simulink model "seldom"  (R2024a)
settings: Solver=FixedStepAuto  StartTime=0.0  StopTime=10.0  FixedStep=framePeriod_s  RelTol=1e-3
undefined symbols (not defined in the file): Aircraft, DiscIntNeverNeededParam, framePeriod_s
libraries: simulink x6, sharedtransform x2, slpidlib x2, matrix_library x1
(part 1 of 2)
settings Model: Creator=brian  LastModifiedBy=joshb
settings SolverCC: AlgebraicLoopSolver=TrustRegion
settings OptimizationCC: DefaultParameterBehavior=Inlined  GainParamInheritBuiltInType=on  UseFloatMulNetSlope=on  DefaultUnderspecifiedDataType=single  StrengthReduction=on  ExpressionFolding=off  BitwiseOrLogicalOp=Bitwise operator  PassReuseOutputArgsAs=Individual arguments  ActiveStateOutputEnumStorageType=uint16  ZeroExternalMemoryAtStartup=off  ZeroInternalMemoryAtStartup=off  EfficientFloat2IntCast=on  LifeSpan=inf  OptimizeBlockOrder=speed  DifferentSizesBufferReuse=on  EfficientTunableParamExpr=on
settings DebuggingCC: ReadBeforeWriteMsg=EnableAllAsError  WriteAfterWriteMsg=EnableAllAsError  WriteAfterReadMsg=EnableAllAsError  IntegerOverflowMsg=error  ParameterPrecisionLossMsg=none  ParameterTunabilityLossMsg=error  UnconnectedInputMsg=warning  UnconnectedOutputMsg=warning  UnconnectedLineMsg=warning  UniqueDataStoreMsg=error  BusObjectLabelMismatch=error  RootOutportRequireBusObject=error  NonBusSignalsTreatedAsBus=error  SFInvalidInputDataAccessInChartInitDiag=error  SFTransitionOutsideNaturalParentDiag=error  SFUnreachableExecutionPathDiag=error  SFUndirectedBroadcastEventsDiag=error  IntegerSaturationMsg=error
settings HardwareCC: ProdBitPerPointer=32  ProdBitPerSizeT=32  ProdBitPerPtrDiffT=32  ProdLargestAtomicInteger=Long  ProdLargestAtomicFloat=Double  ProdWordSize=32  ProdHWDeviceType=NXP->Cortex-M4  TargetBitPerLong=64  TargetBitPerPointer=64  TargetBitPerSizeT=64  TargetBitPerPtrDiffT=64  TargetLargestAtomicFloat=Float  TargetIntDivRoundTo=Zero  TargetEndianess=LittleEndian  TargetWordSize=64  TargetHWDeviceType=Intel->x86-64 (Linux 64)  ProdEqTarget=off
settings ModelReferenceCC: EnableRefExpFcnMdlSchedulingChecks=on  ModelReferenceNumInstancesAllowed=Single
settings SFSimCC: SimParseCustomCode=off  SimGenImportedTypeDefs=on  MATLABDynamicMemAlloc=off  SimTargetLang=C++
settings SFSimCC: SimUserIncludeDirs=|
  | ../../flight_code/include
  | ../../../ua_spaaro_extra/imu/include
  | ../../../ua_spaaro_extra/gnss/include
  | ../../../ua_spaaro_extra/pres/include
  | ../../../ua_spaaro_extra/sbus/include
  | ../../../ua_spaaro_extra/global_defs/include
settings SFSimCC: SimUserDefines=|
  | SIL
  | __FMU_R_V2__
settings RTWCC: Description=Embedded Coder  SystemTargetFile=ert.tlc  GenCodeOnly=on  TemplateMakefile=ert_default_tmf  GenerateReport=on  RTWVerbose=off  RTWUseSimCustomCode=on  Toolchain=GNU gcc/g++ | gmake (64-bit Linux)  BuildConfiguration=Specify  IncludeHyperlinkInReport=on  LaunchReport=on  TargetLang=C++  GenerateTraceInfo=on  GenerateTraceReport=on  GenerateTraceReportSl=on  GenerateTraceReportSf=on  GenerateTraceReportEml=on  GenerateCodeReplacementReport=on  GPUComputeCapability=3.5  DLArmComputeVersion=19.05
settings RTWCC: CustomInclude=|
  | ../../flight_code/include
  | ../../../ua_spaaro_extra/imu/include
  | ../../../ua_spaaro_extra/gnss/include
  | ../../../ua_spaaro_extra/pres/include
  | ../../../ua_spaaro_extra/sbus/include
  | ../../../ua_spaaro_extra/global_defs/include
settings RTWCC: CustomDefine=|
  | SIL
  | __FMU_R_V2__
settings CodeAppCC: ForceParamTrailComments=on  IgnoreCustomStorageClasses=off  OperatorAnnotations=on  SimulinkDataObjDesc=on  SFDataObjDesc=on  MATLABFcnDesc=on  CustomSymbolStrGlobalVar=rt$N$M  CustomSymbolStrType=$N$M  CustomSymbolStrFcn=$N$M$F  CustomSymbolStrMacro=$N$M  InsertBlockDesc=on  StateflowObjectComments=on  MATLABSourceComments=on  EnableCustomComments=on  InternalIdentifier=Classic  InlinedPrmAccess=Macros  ReqsInCode=on
settings ERTTargetCC: TargetLangStandard=C++03 (ISO)  GenerateFullHeader=off  IncludeMdlTerminateFcn=off  CombineSignalStateStructs=on  SuppressErrorStatus=on  SupportAbsoluteTime=off  CodeInterfacePackaging=C++ class  SupportComplex=off  ParenthesesLevel=Standards  CastingMode=Standards  GenerateSharedConstants=off  ERTHeaderFileRootName=autocode$E  ERTSourceFileRootName=autocode$E  RootIOFormat=Structure reference  ERTCustomFileTemplate=example_file_process.tlc  ERTFilePackagingFormat=Compact  PreserveExpressionOrder=on  PreserveIfCondition=on  ConvertIfToSwitch=off  EnableSignedLeftShifts=off  EnableSignedRightShifts=off  IndentSize=4

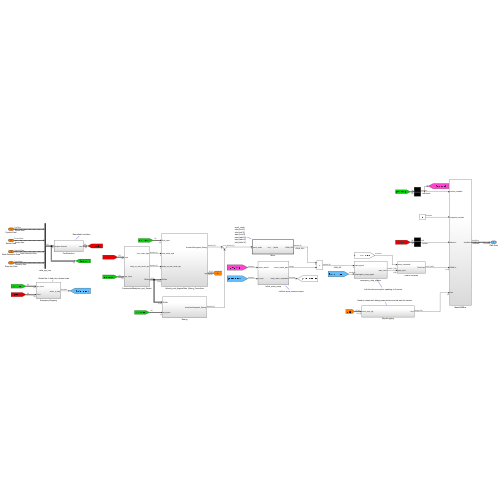
[thumbnail: Simulink's stored preview of the top-level diagram]
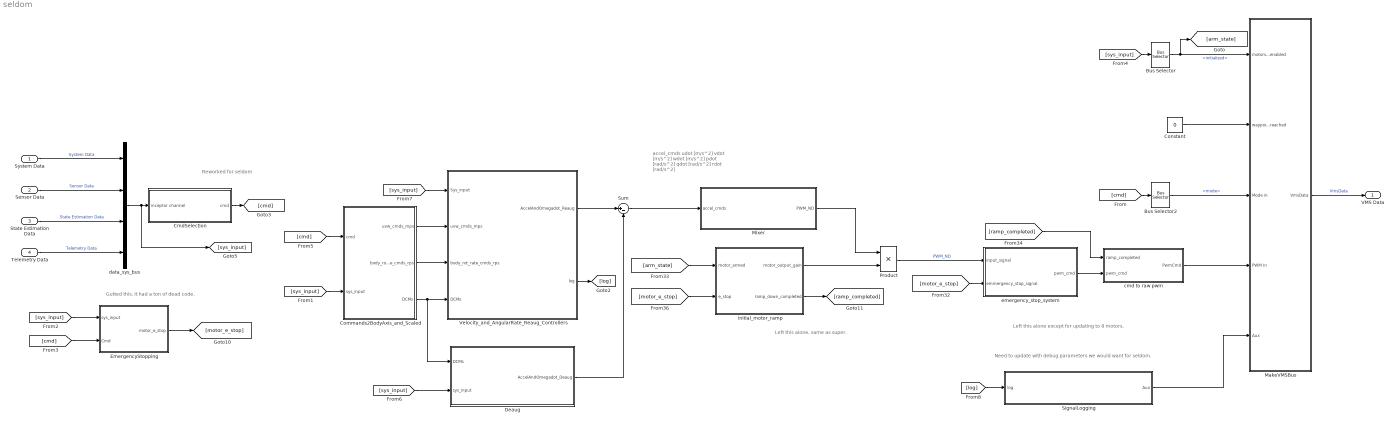
== system seldom ==
  note: accel_cmds
      | udot [m/s^2]
      | vdot [m/s^2]
      | wdot [m/s^2]
      | pdot [rad/s^2]
      | qdot [rad/s^2]
      | rdot [rad/s^2]
  note: Need to update with debug parameters we would want for seldom.
  note: Left this alone, same as super.
  note: Gutted this. It had a ton of dead code.
  note: Reworked for seldom
  note: Left this alone except for updating to 8 motors.
  System Data : Inport  OutDataTypeStr=Bus: SysData  SampleTime=framePeriod_s  BusOutputAsStruct=on
  Sensor Data : Inport  Port=2  OutDataTypeStr=Bus: SensorData  SampleTime=framePeriod_s  BusOutputAsStruct=on
  State Estimation Data : Inport  Port=3  OutDataTypeStr=Bus: StateEstData  SampleTime=framePeriod_s  BusOutputAsStruct=on
  Telemetry Data : Inport  Port=4  OutDataTypeStr=Bus: TelemData  SampleTime=framePeriod_s  BusOutputAsStruct=on
  Bus Selector : BusSelector  OutputSignals=State Estimation Data.bfs_ins.initialized
  Bus Selector2 : BusSelector  OutputSignals=mode
  CmdSelection : Subsystem
  Commands2BodyAxis_and_Scaled : Subsystem
  Constant : Constant  Value=0  OutDataTypeStr=boolean
  Deaug : Subsystem
  EmergencyStopping : Subsystem
  MakeVMSBus : Subsystem
  Mixer : Subsystem
  Product : Product
  SignalLogging : Subsystem
  Sum : Sum  Inputs=|+-
  Velocity_and_AngularRate_Reaug_Controllers : Subsystem
  cmd to raw pwm : Subsystem
  data_sys_bus : BusCreator  Inputs=4
  emergency_stop_system : Subsystem
  initial_motor_ramp : Subsystem
  VMS Data : Outport  OutDataTypeStr=Bus: VmsData  SampleTime=framePeriod_s  BusOutputAsStruct=on
  wires:
  CmdSelection/1(cmd) -> [cmd]
  data_sys_bus/1 -> CmdSelection/1(inceptor channel), [sys_input]
  Velocity_and_AngularRate_Reaug_Controllers/1(AccelAndOmegadot_Reaug) -> Sum/1
  Mixer/1(PWM_ND) -> Product/1
  MakeVMSBus/1(VmsData) -> VMS Data/1  "VmsData"
  cmd to raw pwm/1(PwmCmd) -> MakeVMSBus/4(PWM In)
  [ramp_completed] -> cmd to raw pwm/1(ramp_completed)
  [cmd] -> EmergencyStopping/2(Cmd)
  emergency_stop_system/1(pwm_cmd) -> cmd to raw pwm/2(pwm_cmd)
  [motor_e_stop] -> emergency_stop_system/2(emmergency_stop_signal)
  EmergencyStopping/1(motor_e_stop) -> [motor_e_stop]
  initial_motor_ramp/1(motor_output_gain) -> Product/2
  [motor_e_stop] -> initial_motor_ramp/2(e_stop)
  [arm_state] -> initial_motor_ramp/1(motor_armed)
  Product/1 -> emergency_stop_system/1(input_signal)  "PWM_ND"
  initial_motor_ramp/2(ramp_down_completed) -> [ramp_completed]
  System Data/1 -> data_sys_bus/1  "System Data"
  Sensor Data/1 -> data_sys_bus/2  "Sensor Data"
  Telemetry Data/1 -> data_sys_bus/4  "Telemetry Data"
  [sys_input] -> EmergencyStopping/1(sys_input)
  Bus Selector2/1 -> MakeVMSBus/3(Mode in)  "<mode>"
  Constant/1 -> MakeVMSBus/2(waypoint_reached)
  Bus Selector/1 -> MakeVMSBus/1(motors_enabled), [arm_state]  "<initialized>"
  State Estimation Data/1 -> data_sys_bus/3  "State Estimation Data"
  [sys_input] -> Bus Selector/1
  [cmd] -> Bus Selector2/1
  SignalLogging/1(Aux) -> MakeVMSBus/5(Aux)
  Sum/1 -> Mixer/1(accel_cmds)
  [cmd] -> Commands2BodyAxis_and_Scaled/1(cmd)
  [sys_input] -> Commands2BodyAxis_and_Scaled/2(sys_input)
  Commands2BodyAxis_and_Scaled/3(DCMs) -> Deaug/1(DCMs), Velocity_and_AngularRate_Reaug_Controllers/4(DCMs)
  [sys_input] -> Deaug/2(sys_input)
  Deaug/1(AccelAndOmegadot_Deaug) -> Sum/2
  [sys_input] -> Velocity_and_AngularRate_Reaug_Controllers/1(Sys_input)
  Commands2BodyAxis_and_Scaled/1(uvw_cmds_mps) -> Velocity_and_AngularRate_Reaug_Controllers/2(uvw_cmds_mps)
  Commands2BodyAxis_and_Scaled/2(body_rot_rate_cmds_rps) -> Velocity_and_AngularRate_Reaug_Controllers/3(body_rot_rate_cmds_rps)
  Velocity_and_AngularRate_Reaug_Controllers/2(log) -> [log]
  [log] -> SignalLogging/1(log)

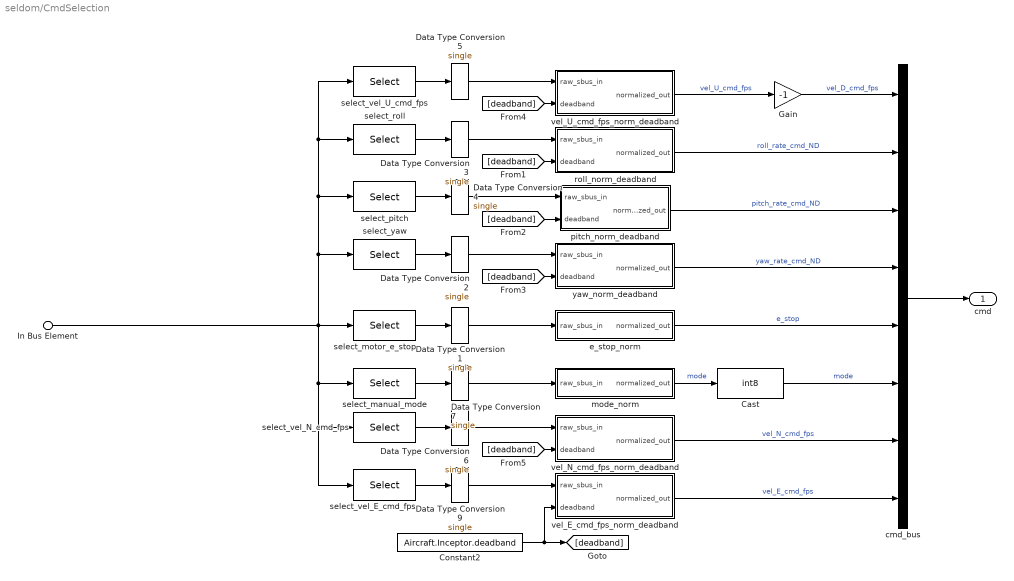
== system seldom/CmdSelection ==
  In Bus Element : Inport  PortName=inceptor channel  Element=Sensor Data.inceptor.ch
  Cast : DataTypeConversion  OutDataTypeStr=int8  SaturateOnIntegerOverflow=off  RndMeth=Floor
  Constant2 : Constant  Value=Aircraft.Inceptor.deadband
  Data Type Conversion{1..7,9} (8 alike) : DataTypeConversion  OutDataTypeStr=single  SaturateOnIntegerOverflow=off  RndMeth=Floor
  Gain : Gain  Gain=-1
  cmd_bus : BusCreator  Inputs=8
  e_stop_norm : Subsystem
  mode_norm : Subsystem
  pitch_norm_deadband : Subsystem
  roll_norm_deadband : Subsystem
  select_manual_mode : Selector  IndexOptions=Index vector (dialog)  Indices=Aircraft.Inceptor.mode  OutputSizes=1
  select_motor_e_stop : Selector  IndexOptions=Index vector (dialog)  Indices=Aircraft.Inceptor.throttle_e_stop  OutputSizes=1
  select_pitch : Selector  IndexOptions=Index vector (dialog)  Indices=Aircraft.Inceptor.pitch_rate  OutputSizes=1
  select_roll : Selector  IndexOptions=Index vector (dialog)  Indices=Aircraft.Inceptor.roll_rate  OutputSizes=1
  select_vel_E_cmd_fps : Selector  IndexOptions=Index vector (dialog)  Indices=Aircraft.Inceptor.vel_E_cmd_fps  OutputSizes=1
  select_vel_N_cmd_fps : Selector  IndexOptions=Index vector (dialog)  Indices=Aircraft.Inceptor.vel_N_cmd_fps  OutputSizes=1
  select_vel_U_cmd_fps : Selector  IndexOptions=Index vector (dialog)  Indices=Aircraft.Inceptor.vel_U_cmd_fps  OutputSizes=1
  select_yaw : Selector  IndexOptions=Index vector (dialog)  Indices=Aircraft.Inceptor.yaw_rate  OutputSizes=1
  vel_E_cmd_fps_norm_deadband : Subsystem
  vel_N_cmd_fps_norm_deadband : Subsystem
  vel_U_cmd_fps_norm_deadband : Subsystem
  yaw_norm_deadband : Subsystem
  cmd : Outport
  wires:
  select_pitch/1 -> Data Type Conversion4/1
  select_yaw/1 -> Data Type Conversion2/1
  Data Type Conversion2/1 -> yaw_norm_deadband/1(raw_sbus_in)
  select_vel_U_cmd_fps/1 -> Data Type Conversion5/1
  Data Type Conversion4/1 -> pitch_norm_deadband/1(raw_sbus_in)
  cmd_bus/1 -> cmd/1
  Data Type Conversion3/1 -> roll_norm_deadband/1(raw_sbus_in)
  Data Type Conversion5/1 -> vel_U_cmd_fps_norm_deadband/1(raw_sbus_in)
  select_roll/1 -> Data Type Conversion3/1
  In Bus Element/1 -> select_vel_E_cmd_fps/1, select_vel_N_cmd_fps/1, select_manual_mode/1, select_vel_U_cmd_fps/1, select_roll/1, select_pitch/1, select_yaw/1, select_motor_e_stop/1
  Data Type Conversion1/1 -> e_stop_norm/1(raw_sbus_in)
  select_motor_e_stop/1 -> Data Type Conversion1/1
  select_vel_N_cmd_fps/1 -> Data Type Conversion6/1
  Data Type Conversion6/1 -> vel_N_cmd_fps_norm_deadband/1(raw_sbus_in)
  Data Type Conversion7/1 -> mode_norm/1(raw_sbus_in)
  select_manual_mode/1 -> Data Type Conversion7/1
  select_vel_E_cmd_fps/1 -> Data Type Conversion9/1
  Data Type Conversion9/1 -> vel_E_cmd_fps_norm_deadband/1(raw_sbus_in)
  Gain/1 -> cmd_bus/1  "vel_D_cmd_fps"
  pitch_norm_deadband/1(normalized_out) -> cmd_bus/3  "pitch_rate_cmd_ND"
  roll_norm_deadband/1(normalized_out) -> cmd_bus/2  "roll_rate_cmd_ND"
  yaw_norm_deadband/1(normalized_out) -> cmd_bus/4  "yaw_rate_cmd_ND"
  e_stop_norm/1(normalized_out) -> cmd_bus/5  "e_stop"
  mode_norm/1(normalized_out) -> Cast/1  "mode"
  vel_N_cmd_fps_norm_deadband/1(normalized_out) -> cmd_bus/7  "vel_N_cmd_fps"
  vel_E_cmd_fps_norm_deadband/1(normalized_out) -> cmd_bus/8  "vel_E_cmd_fps"
  [deadband] -> roll_norm_deadband/2(deadband)
  [deadband] -> vel_U_cmd_fps_norm_deadband/2(deadband)
  [deadband] -> pitch_norm_deadband/2(deadband)
  [deadband] -> yaw_norm_deadband/2(deadband)
  [deadband] -> vel_N_cmd_fps_norm_deadband/2(deadband)
  Constant2/1 -> vel_E_cmd_fps_norm_deadband/2(deadband), [deadband]
  vel_U_cmd_fps_norm_deadband/1(normalized_out) -> Gain/1  "vel_U_cmd_fps"
  Cast/1 -> cmd_bus/6  "mode"

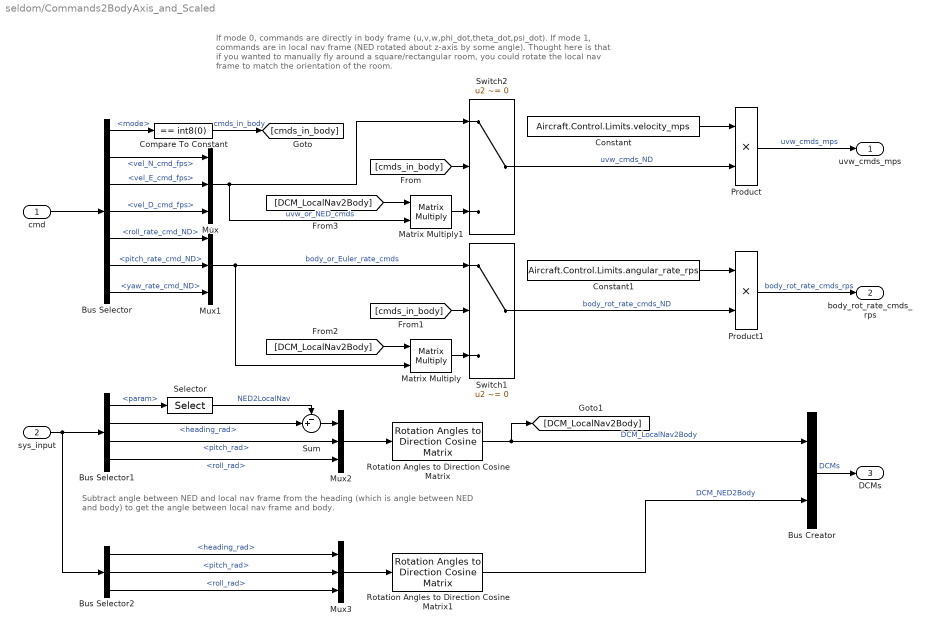
== system seldom/Commands2BodyAxis_and_Scaled ==
  note: Subtract angle between NED and local nav frame from the heading (which is angle between NED and body) to get the angle between local nav frame and body.
  note: If mode 0, commands are directly in body frame (u,v,w,phi_dot,theta_dot,psi_dot).
      | If mode 1, commands are in local nav frame (NED rotated about z-axis by some angle).
      |     Thought here is that if you wanted to manually fly around a square/rectangular room, you could rotate the local nav frame to match the orientation of the room.
  cmd : Inport
  sys_input : Inport  Port=2
  Bus Creator : BusCreator  Inputs=2
  Bus Selector : BusSelector  OutputSignals=mode,vel_N_cmd_fps,vel_E_cmd_fps,vel_D_cmd_fps,roll_rate_cmd_ND,pitch_rate_cmd_ND,yaw_rate_cmd_ND
  Bus Selector1 : BusSelector  OutputSignals=Telemetry Data.param,State Estimation Data.bfs_ins.heading_rad,State Estimation Data.bfs_ins.pitch_rad,State Estimation Data.bfs_ins.roll_rad
  Bus Selector2 : BusSelector  OutputSignals=State Estimation Data.bfs_ins.heading_rad,State Estimation Data.bfs_ins.pitch_rad,State Estimation Data.bfs_ins.roll_rad
  Compare To Constant : simulink/Logic and Bit Operations/Compare To Constant  relop===  const=int8(0)  OutDataTypeStr=boolean
  Constant : Constant  Value=Aircraft.Control.Limits.velocity_mps
  Constant1 : Constant  Value=Aircraft.Control.Limits.angular_rate_rps
  Matrix Multiply : Product  Multiplication=Matrix(*)
  Matrix Multiply1 : Product  Multiplication=Matrix(*)
  Mux{,1..3} (4 alike) : Mux  Inputs=3
  Product : Product
  Product1 : Product
  Rotation Angles to Direction Cosine Matrix : sharedtransform/Rotation Angles to Direction Cosine Matrix  rotationOrder=ZYX  aMode=aMode
  Rotation Angles to Direction Cosine Matrix1 : sharedtransform/Rotation Angles to Direction Cosine Matrix  rotationOrder=ZYX  aMode=aMode
  Selector : Selector  InputPortWidth=24  IndexOptions=Index vector (dialog)  Indices=[1]  OutputSizes=1
  Sum : Sum  Inputs=-+|
  Switch1 : Switch  Criteria=u2 ~= 0  SaturateOnIntegerOverflow=off  InputSameDT=off
  Switch2 : Switch  Criteria=u2 ~= 0  SaturateOnIntegerOverflow=off  InputSameDT=off
  uvw_cmds_mps : Outport
  body_rot_rate_cmds_rps : Outport  Port=2
  DCMs : Outport  Port=3
  wires:
  cmd/1 -> Bus Selector/1
  Bus Selector/1 -> Compare To Constant/1  "<mode>"
  Bus Selector/2 -> Mux/1  "<vel_N_cmd_fps>"
  Bus Selector/3 -> Mux/2  "<vel_E_cmd_fps>"
  Bus Selector/4 -> Mux/3  "<vel_D_cmd_fps>"
  Mux/1 -> Switch2/1, Matrix Multiply1/2  "uvw_or_NED_cmds"
  Bus Selector/5 -> Mux1/1  "<roll_rate_cmd_ND>"
  Bus Selector/6 -> Mux1/2  "<pitch_rate_cmd_ND>"
  Bus Selector/7 -> Mux1/3  "<yaw_rate_cmd_ND>"
  Mux1/1 -> Matrix Multiply/2, Switch1/1  "body_or_Euler_rate_cmds"
  Rotation Angles to Direction Cosine Matrix/1 -> Bus Creator/1, [DCM_LocalNav2Body]  "DCM_LocalNav2Body"
  sys_input/1 -> Bus Selector2/1, Bus Selector1/1
  Bus Selector1/2 -> Sum/2  "<heading_rad>"
  Bus Selector1/3 -> Mux2/2  "<pitch_rad>"
  Bus Selector1/4 -> Mux2/3  "<roll_rad>"
  Mux2/1 -> Rotation Angles to Direction Cosine Matrix/1
  Bus Selector1/1 -> Selector/1  "<param>"
  Selector/1 -> Sum/1  "NED2LocalNav"
  Sum/1 -> Mux2/1
  Compare To Constant/1 -> [cmds_in_body]  "cmds_in_body"
  [cmds_in_body] -> Switch2/2
  [cmds_in_body] -> Switch1/2
  [DCM_LocalNav2Body] -> Matrix Multiply/1
  Matrix Multiply/1 -> Switch1/3
  Matrix Multiply1/1 -> Switch2/3
  [DCM_LocalNav2Body] -> Matrix Multiply1/1
  Switch2/1 -> Product/2  "uvw_cmds_ND"
  Switch1/1 -> Product1/2  "body_rot_rate_cmds_ND"
  Product/1 -> uvw_cmds_mps/1  "uvw_cmds_mps"
  Constant/1 -> Product/1
  Product1/1 -> body_rot_rate_cmds_rps/1  "body_rot_rate_cmds_rps"
  Constant1/1 -> Product1/1
  Mux3/1 -> Rotation Angles to Direction Cosine Matrix1/1
  Bus Selector2/1 -> Mux3/1  "<heading_rad>"
  Bus Selector2/2 -> Mux3/2  "<pitch_rad>"
  Bus Selector2/3 -> Mux3/3  "<roll_rad>"
  Rotation Angles to Direction Cosine Matrix1/1 -> Bus Creator/2  "DCM_NED2Body"
  Bus Creator/1 -> DCMs/1  "DCMs"

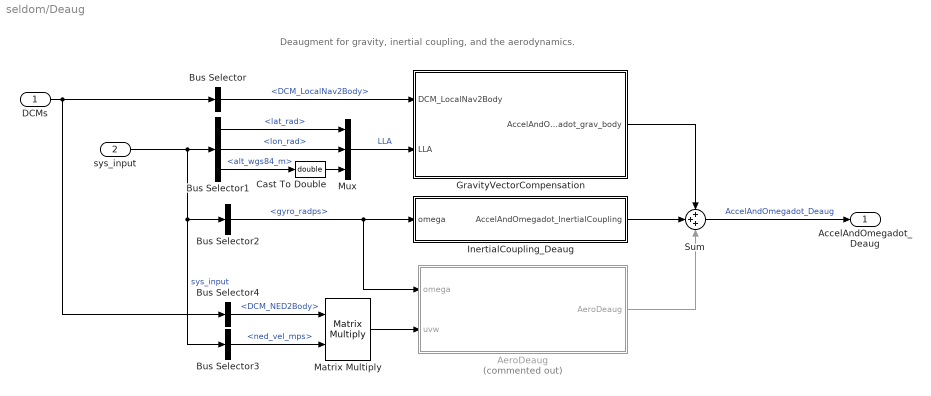
== system seldom/Deaug ==
  note: Deaugment for gravity, inertial coupling, and the aerodynamics.
  DCMs : Inport
  sys_input : Inport  Port=2
  AeroDeaug : Subsystem  Commented=on
  Bus Selector : BusSelector  OutputSignals=DCM_LocalNav2Body
  Bus Selector1 : BusSelector  OutputSignals=Sensor Data.ext_gnss1.lat_rad,Sensor Data.ext_gnss1.lon_rad,Sensor Data.ext_gnss1.alt_wgs84_m
  Bus Selector2 : BusSelector  OutputSignals=Sensor Data.fmu_imu.gyro_radps
  Bus Selector3 : BusSelector  OutputSignals=State Estimation Data.bfs_ins.ned_vel_mps
  Bus Selector4 : BusSelector  OutputSignals=DCM_NED2Body
  Cast To Double : DataTypeConversion  OutDataTypeStr=double  SaturateOnIntegerOverflow=off  RndMeth=Floor
  GravityVectorCompensation : Subsystem
  InertialCoupling_Deaug : Subsystem
  Matrix Multiply : Product  Multiplication=Matrix(*)
  Mux : Mux  Inputs=3
  Sum : Sum  Inputs=+++
  AccelAndOmegadot_Deaug : Outport
  wires:
  Bus Selector1/2 -> Mux/2  "<lon_rad>"
  Bus Selector/1 -> GravityVectorCompensation/1(DCM_LocalNav2Body)  "<DCM_LocalNav2Body>"
  sys_input/1 -> Bus Selector1/1, Bus Selector2/1, Bus Selector3/1  "sys_input"
  Bus Selector1/3 -> Cast To Double/1  "<alt_wgs84_m>"
  GravityVectorCompensation/1(AccelAndOmegadot_grav_body) -> Sum/1
  Mux/1 -> GravityVectorCompensation/2(LLA)  "LLA"
  InertialCoupling_Deaug/1(AccelAndOmegadot_InertialCoupling) -> Sum/2
  Bus Selector1/1 -> Mux/1  "<lat_rad>"
  Bus Selector2/1 -> AeroDeaug/1(omega), InertialCoupling_Deaug/1(omega)  "<gyro_radps>"
  Bus Selector3/1 -> Matrix Multiply/2  "<ned_vel_mps>"
  Bus Selector4/1 -> Matrix Multiply/1  "<DCM_NED2Body>"
  Matrix Multiply/1 -> AeroDeaug/2(uvw)
  AeroDeaug/1(AeroDeaug) -> Sum/3
  Sum/1 -> AccelAndOmegadot_Deaug/1  "AccelAndOmegadot_Deaug"
  Cast To Double/1 -> Mux/3
  DCMs/1 -> Bus Selector4/1, Bus Selector/1

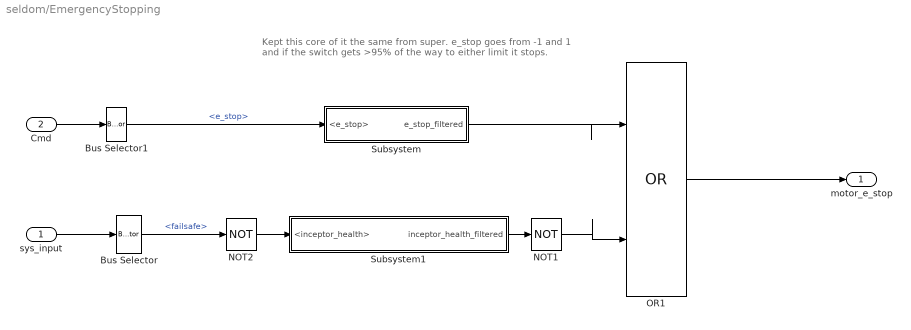
== system seldom/EmergencyStopping ==
  note: Kept this core of it the same from super. e_stop goes from -1 and 1 and if the switch gets >95% of the way to either limit it stops.
  sys_input : Inport
  Cmd : Inport  Port=2
  Bus Selector : BusSelector  OutputSignals=Sensor Data.inceptor.failsafe
  Bus Selector1 : BusSelector  OutputSignals=e_stop
  NOT1 : Logic  Operator=NOT  IconShape=distinctive  AllPortsSameDT=off  OutDataTypeStr=boolean
  NOT2 : Logic  Operator=NOT  IconShape=distinctive  AllPortsSameDT=off  OutDataTypeStr=boolean
  OR1 : Logic  Operator=OR  IconShape=distinctive  AllPortsSameDT=off  OutDataTypeStr=boolean
  Subsystem : Subsystem
  Subsystem1 : Subsystem
  motor_e_stop : Outport
  wires:
  Bus Selector/1 -> NOT2/1  "<failsafe>"
  sys_input/1 -> Bus Selector/1
  Bus Selector1/1 -> Subsystem/1(<e_stop>)  "<e_stop>"
  Cmd/1 -> Bus Selector1/1
  OR1/1 -> motor_e_stop/1
  NOT1/1 -> OR1/2
  Subsystem/1(e_stop_filtered) -> OR1/1
  NOT2/1 -> Subsystem1/1(<inceptor_health>)
  Subsystem1/1(inceptor_health_filtered) -> NOT1/1

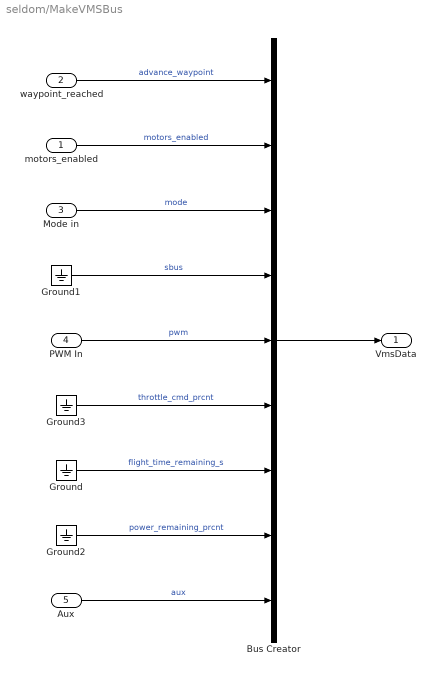
== system seldom/MakeVMSBus ==
  motors_enabled : Inport
  waypoint_reached : Inport  Port=2
  Mode in : Inport  Port=3
  PWM In : Inport  Port=4
  Aux : Inport  Port=5
  Bus Creator : BusCreator  Inputs=9  OutDataTypeStr=Bus: VmsData  NonVirtualBus=on
      settings: InheritFromInputs=off
  Ground{,1..3} (4 alike) : Ground
  VmsData : Outport
  wires:
  Bus Creator/1 -> VmsData/1
  waypoint_reached/1 -> Bus Creator/1  "advance_waypoint"
  motors_enabled/1 -> Bus Creator/2  "motors_enabled"
  Mode in/1 -> Bus Creator/3  "mode"
  Ground1/1 -> Bus Creator/4  "sbus"
  PWM In/1 -> Bus Creator/5  "pwm"
  Ground3/1 -> Bus Creator/6  "throttle_cmd_prcnt"
  Aux/1 -> Bus Creator/9  "aux"
  Ground/1 -> Bus Creator/7  "flight_time_remaining_s"
  Ground2/1 -> Bus Creator/8  "power_remaining_prcnt"

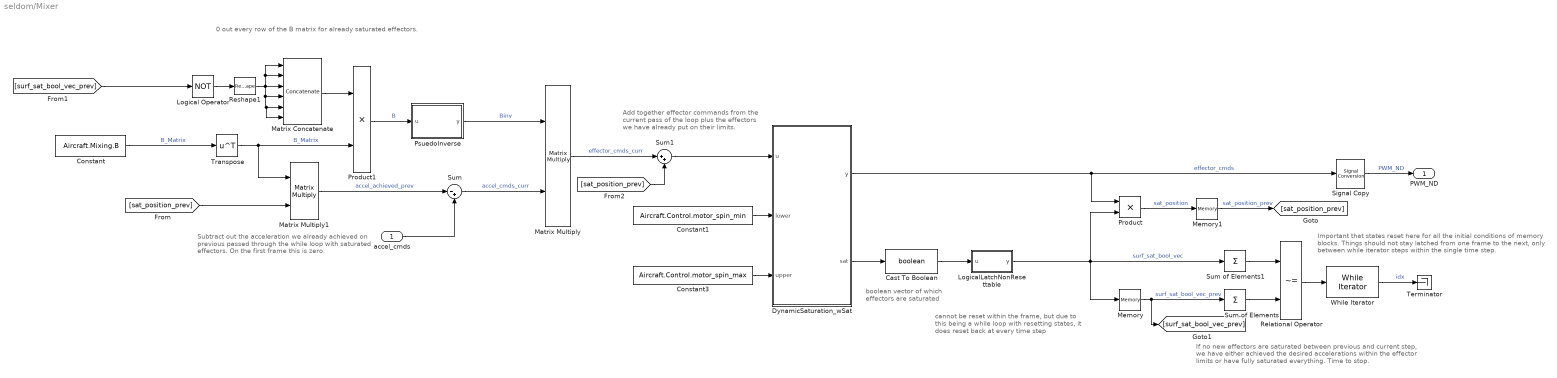
== system seldom/Mixer ==
  note: Add together effector commands from the current pass of the loop plus the effectors we have already put on their limits.
  note: Subtract out the acceleration we already achieved on previous passed through the while loop with saturated effectors. On the first frame this is zero.
  note: 0 out every row of the B matrix for already saturated effectors.
  note: Important that states reset here for all the initial conditions of memory blocks. Things should not stay latched from one frame to the next, only between while iterator steps within the single time step.
  note: If no new effectors are saturated between previous and current step, we have either achieved the desired accelerations within the effector limits or have fully saturated everything. Time to stop.
  note: cannot be reset within the frame, but due to this being a while loop with resetting states, it does reset back at every time step
  note: boolean vector of which effectors are saturated
  accel_cmds : Inport
  Cast To Boolean : DataTypeConversion  OutDataTypeStr=boolean  SaturateOnIntegerOverflow=off  RndMeth=Floor
  Constant : Constant  Value=Aircraft.Mixing.B
  Constant1 : Constant  Value=Aircraft.Control.motor_spin_min  OutDataTypeStr=single
  Constant3 : Constant  Value=Aircraft.Control.motor_spin_max  OutDataTypeStr=single
  DynamicSaturation_wSat : Subsystem
  Logical Operator : Logic  Operator=NOT  AllPortsSameDT=off  OutDataTypeStr=boolean
  LogicalLatchNonResettable : Subsystem
  Matrix Concatenate : Concatenate  NumInputs=6  Mode=Multidimensional array
  Matrix Multiply : Product  Multiplication=Matrix(*)
  Matrix Multiply1 : Product  Multiplication=Matrix(*)
  Memory : Memory  InitialCondition=zeros(1,Aircraft.Motor.nMotor)  InheritSampleTime=on
  Memory1 : Memory  InitialCondition=zeros(1,Aircraft.Motor.nMotor)  InheritSampleTime=on
  Product : Product
  Product1 : Product
  PsuedoInverse : MATLAB Function  TreatAsAtomicUnit=on
  Relational Operator : RelationalOperator  Operator=~=  OutDataTypeStr=boolean  RndMeth=Simplest  InputSameDT=off
  Reshape1 : Reshape  OutputDimensionality=Row vector (2-D)
  Signal Copy : SignalConversion  OverrideOpt=off
  Sum : Sum  Inputs=|-+
  Sum of Elements : Sum  Inputs=+
  Sum of Elements1 : Sum  Inputs=+
  Sum1 : Sum  Inputs=|++
  Terminator : Terminator
  Transpose : Math  Operator=transpose
  While Iterator : WhileIterator  WhileBlockType=do-while  ResetStates=reset  ShowIterationPort=on
  PWM_ND : Outport
  wires:
  Constant/1 -> Transpose/1  "B_Matrix"
  accel_cmds/1 -> Sum/2
  DynamicSaturation_wSat/1(y) -> Product/1, Signal Copy/1  "effector_cmds"
  Constant3/1 -> DynamicSaturation_wSat/3(upper)
  Constant1/1 -> DynamicSaturation_wSat/2(lower)
  Sum1/1 -> DynamicSaturation_wSat/1(u)
  DynamicSaturation_wSat/2(sat) -> Cast To Boolean/1
  Cast To Boolean/1 -> LogicalLatchNonResettable/1(u)
  LogicalLatchNonResettable/1(y) -> Product/2, Sum of Elements1/1, Memory/1  "surf_sat_bool_vec"
  Memory/1 -> Sum of Elements/1, [surf_sat_bool_vec_prev]  "surf_sat_bool_vec_prev"
  Sum of Elements/1 -> Relational Operator/2
  Sum of Elements1/1 -> Relational Operator/1
  Relational Operator/1 -> While Iterator/1
  While Iterator/1 -> Terminator/1  "idx"
  Product/1 -> Memory1/1  "sat_position"
  Memory1/1 -> [sat_position_prev]  "sat_position_prev"
  [sat_position_prev] -> Matrix Multiply1/2
  [surf_sat_bool_vec_prev] -> Logical Operator/1
  Logical Operator/1 -> Reshape1/1
  Reshape1/1 -> Matrix Concatenate/6, Matrix Concatenate/5, Matrix Concatenate/4, Matrix Concatenate/1, Matrix Concatenate/2, Matrix Concatenate/3
  Matrix Concatenate/1 -> Product1/1
  Transpose/1 -> Product1/2, Matrix Multiply1/1  "B_Matrix"
  Product1/1 -> PsuedoInverse/1(u)  "B"
  PsuedoInverse/1(y) -> Matrix Multiply/1  "Binv"
  Matrix Multiply1/1 -> Sum/1  "accel_achieved_prev"
  Sum/1 -> Matrix Multiply/2  "accel_cmds_curr"
  Matrix Multiply/1 -> Sum1/1  "effector_cmds_curr"
  [sat_position_prev] -> Sum1/2
  Signal Copy/1 -> PWM_ND/1  "PWM_ND"

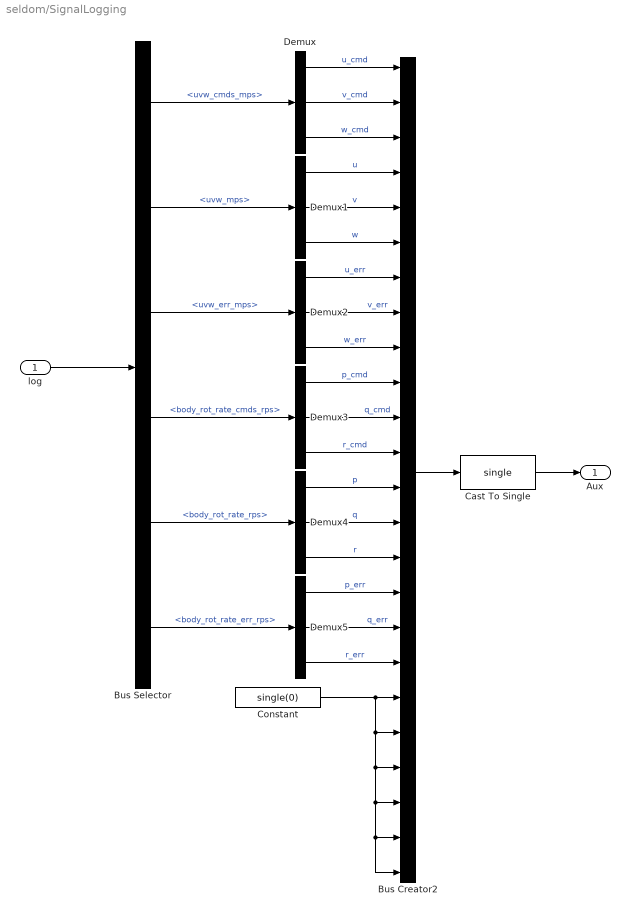
== system seldom/SignalLogging ==
  log : Inport
  Bus Creator2 : BusCreator  Inputs=24
  Bus Selector : BusSelector  OutputSignals=uvw_cmds_mps,uvw_mps,uvw_err_mps,body_rot_rate_cmds_rps,body_rot_rate_rps,body_rot_rate_err_rps
  Cast To Single : DataTypeConversion  OutDataTypeStr=single  SaturateOnIntegerOverflow=off  RndMeth=Floor
  Constant : Constant  Value=single(0)
  Demux{,1..5} (6 alike) : Demux  Outputs=3
  Aux : Outport
  wires:
  Cast To Single/1 -> Aux/1
  Bus Creator2/1 -> Cast To Single/1
  log/1 -> Bus Selector/1
  Bus Selector/6 -> Demux5/1  "<body_rot_rate_err_rps>"
  Demux/1 -> Bus Creator2/1  "u_cmd"
  Demux/2 -> Bus Creator2/2  "v_cmd"
  Demux/3 -> Bus Creator2/3  "w_cmd"
  Demux1/1 -> Bus Creator2/4  "u"
  Demux1/2 -> Bus Creator2/5  "v"
  Demux1/3 -> Bus Creator2/6  "w"
  Demux2/1 -> Bus Creator2/7  "u_err"
  Demux2/2 -> Bus Creator2/8  "v_err"
  Demux2/3 -> Bus Creator2/9  "w_err"
  Demux5/3 -> Bus Creator2/18  "r_err"
  Demux5/2 -> Bus Creator2/17  "q_err"
  Demux5/1 -> Bus Creator2/16  "p_err"
  Demux4/3 -> Bus Creator2/15  "r"
  Demux4/2 -> Bus Creator2/14  "q"
  Demux4/1 -> Bus Creator2/13  "p"
  Demux3/3 -> Bus Creator2/12  "r_cmd"
  Demux3/2 -> Bus Creator2/11  "q_cmd"
  Demux3/1 -> Bus Creator2/10  "p_cmd"
  Bus Selector/2 -> Demux1/1  "<uvw_mps>"
  Bus Selector/1 -> Demux/1  "<uvw_cmds_mps>"
  Bus Selector/3 -> Demux2/1  "<uvw_err_mps>"
  Bus Selector/4 -> Demux3/1  "<body_rot_rate_cmds_rps>"
  Bus Selector/5 -> Demux4/1  "<body_rot_rate_rps>"
  Constant/1 -> Bus Creator2/20, Bus Creator2/21, Bus Creator2/23, Bus Creator2/24, Bus Creator2/22, Bus Creator2/19

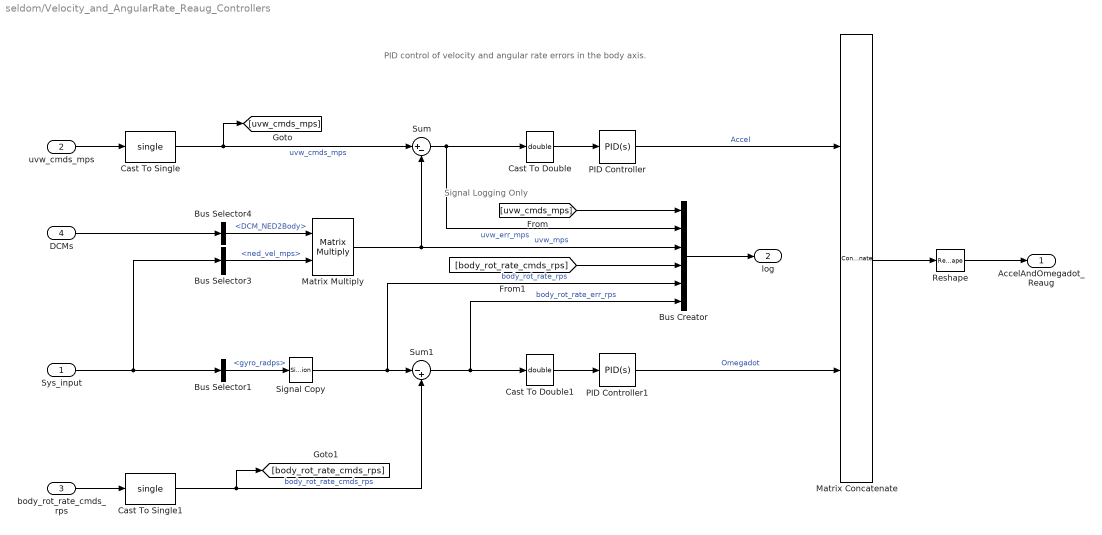
== system seldom/Velocity_and_AngularRate_Reaug_Controllers ==
  note: PID control of velocity and angular rate errors in the body axis.
  note: Signal Logging Only
  Sys_input : Inport
  uvw_cmds_mps : Inport  Port=2
  body_rot_rate_cmds_rps : Inport  Port=3
  DCMs : Inport  Port=4
  Bus Creator : BusCreator  Inputs=6
  Bus Selector1 : BusSelector  OutputSignals=Sensor Data.fmu_imu.gyro_radps
  Bus Selector3 : BusSelector  OutputSignals=State Estimation Data.bfs_ins.ned_vel_mps
  Bus Selector4 : BusSelector  OutputSignals=DCM_NED2Body
  Cast To Double : DataTypeConversion  OutDataTypeStr=double  SaturateOnIntegerOverflow=off  RndMeth=Floor
  Cast To Double1 : DataTypeConversion  OutDataTypeStr=double  SaturateOnIntegerOverflow=off  RndMeth=Floor
  Cast To Single : DataTypeConversion  OutDataTypeStr=single  SaturateOnIntegerOverflow=off  RndMeth=Floor
  Cast To Single1 : DataTypeConversion  OutDataTypeStr=single  SaturateOnIntegerOverflow=off  RndMeth=Floor
  Matrix Concatenate : Concatenate  Mode=Multidimensional array
  Matrix Multiply : Product  Multiplication=Matrix(*)
  PID Controller : slpidlib/PID Controller  Controller=PID  Form=Parallel  TimeDomain=Continuous-time  UseExternalTs=off  SampleTime=-1  IntegratorMethod=Forward Euler  FilterMethod=Forward Euler  ControllerParametersSource=internal  P=1  I=.1  UseKiTs=off  D=.3  UseExternalDerivativeSource=off  N=100  UseFilter=on  TunerSelectOption=Transfer Function Based (PID Tuner App)  InitialConditionSource=internal  InitialConditionForIntegrator=0  InitialConditionForFilter=0  DifferentiatorICPrevScaledInput=0  ExternalReset=none  TrackingMode=off  Kt=1  LimitOutput=off  SatLimitsSource=internal  UpperSaturationLimit=inf  LowerSaturationLimit=-inf  LinearizeAsGain=on  AntiWindupMode=none  Kb=1  LimitIntegrator=off  UpperIntegratorSaturationLimit=inf  LowerIntegratorSaturationLimit=-inf  POutMin=[]  POutMax=[]  IOutMin=[]  IOutMax=[]  DOutMin=[]  DOutMax=[]  NOutMin=[]  NOutMax=[]  SumOutMin=[]  SumOutMax=[]  SaturationOutMin=[]  SaturationOutMax=[]  PParamMin=[]  PParamMax=[]  IParamMin=[]  IParamMax=[]  DParamMin=[]  DParamMax=[]  NParamMin=[]  NParamMax=[]  KbParamMin=[]  KbParamMax=[]  KtParamMin=[]  KtParamMax=[]  KbOutMin=[]  KbOutMax=[]  KtOutMin=[]  KtOutMax=[]  IntegratorOutMin=[]  IntegratorOutMax=[]  FilterOutMin=[]  FilterOutMax=[]  SumI1OutMin=[]  SumI1OutMax=[]  SumI2OutMin=[]  SumI2OutMax=[]  SumI3OutMin=[]  SumI3OutMax=[]  SumI4OutMin=[]  SumI4OutMax=[]  SumDOutMin=[]  SumDOutMax=[]  DifferentiatorOutMin=[]  DifferentiatorOutMax=[]  FilterDiffOutCoefMin=[]  FilterDiffOutCoefMax=[]  ReciprocalOutMin=[]  ReciprocalOutMax=[]  SumDenOutMin=[]  SumDenOutMax=[]  SumNumOutMin=[]  SumNumOutMax=[]  DivideOutMin=[]  DivideOutMax=[]  UdiffTsProdOutMin=[]  UdiffTsProdOutMax=[]  NTsProdOutMin=[]  NTsProdOutMax=[]  UintegralTsProdOutMin=[]  UintegralTsProdOutMax=[]  UngainTsProdOutMin=[]  UngainTsProdOutMax=[]  ClampingZeroOutDataTypeStr=Inherit: Inherit via back propagation  ClampingZeroOutMin=[]  ClampingZeroOutMax=[]  FilterDenConstantOutDataTypeStr=Inherit: Inherit via back propagation  FilterDenConstantOutMin=[]  FilterDenConstantOutMax=[]  PCopyOutDataTypeStr=Inherit: Inherit via back propagation  PCopyOutMin=[]  PCopyOutMax=[]  NCopyOutDataTypeStr=Inherit: Inherit via back propagation  NCopyOutMin=[]  NCopyOutMax=[]  IntegratorContinuousStateAttributes=''  IntegratorStateMustResolveToSignalObject=off  IntegratorRTWStateStorageClass=Auto  FilterContinuousStateAttributes=''  FilterStateMustResolveToSignalObject=off  FilterRTWStateStorageClass=Auto  ParallelPVariant=InternalParameters  IdealPVariant=Disabled  IVariant=InternalParameters  DVariant=InternalParameters  IntegratorVariant=Continuous  SatVariant=Disabled  AWVariant=Passthrough  PCopyVariant=Disabled  TRVariant=Disabled  FdbkBlocksVariant=Forward  IdealPFdbkVariant=Disabled  SatFdbkVariant=Disabled  DerivativeFilterVariant=ContFilter  NVariant=InternalParameters  NCopyVariant=Disabled  FilterICVariant=InternalICsFilter  IntegratorICVariant=InternalICs  ExternalResetVariant=Disabled  TRSumVariant=Passthrough  SumFdbkVariant=Disabled  SumVariant=Sum_PID  TsampFilterVariant=InternalTs  TsampNgainVariant=Passthrough  TsampIntegralVariant=Disabled_SignalSpec  ExternalSaturationOutDataTypeStr=Inherit: Same as second input  DerivativeSourceVariant=ErrorSignal
  PID Controller1 : slpidlib/PID Controller  Controller=PID  Form=Parallel  TimeDomain=Continuous-time  UseExternalTs=off  SampleTime=-1  IntegratorMethod=Forward Euler  FilterMethod=Forward Euler  ControllerParametersSource=internal  P=.5  I=.05  UseKiTs=off  D=.15  UseExternalDerivativeSource=off  N=100  UseFilter=on  TunerSelectOption=Transfer Function Based (PID Tuner App)  InitialConditionSource=internal  InitialConditionForIntegrator=0  InitialConditionForFilter=0  DifferentiatorICPrevScaledInput=0  ExternalReset=none  TrackingMode=off  Kt=1  LimitOutput=off  SatLimitsSource=internal  UpperSaturationLimit=inf  LowerSaturationLimit=-inf  LinearizeAsGain=on  AntiWindupMode=none  Kb=1  LimitIntegrator=off  UpperIntegratorSaturationLimit=inf  LowerIntegratorSaturationLimit=-inf  POutMin=[]  POutMax=[]  IOutMin=[]  IOutMax=[]  DOutMin=[]  DOutMax=[]  NOutMin=[]  NOutMax=[]  SumOutMin=[]  SumOutMax=[]  SaturationOutMin=[]  SaturationOutMax=[]  PParamMin=[]  PParamMax=[]  IParamMin=[]  IParamMax=[]  DParamMin=[]  DParamMax=[]  NParamMin=[]  NParamMax=[]  KbParamMin=[]  KbParamMax=[]  KtParamMin=[]  KtParamMax=[]  KbOutMin=[]  KbOutMax=[]  KtOutMin=[]  KtOutMax=[]  IntegratorOutMin=[]  IntegratorOutMax=[]  FilterOutMin=[]  FilterOutMax=[]  SumI1OutMin=[]  SumI1OutMax=[]  SumI2OutMin=[]  SumI2OutMax=[]  SumI3OutMin=[]  SumI3OutMax=[]  SumI4OutMin=[]  SumI4OutMax=[]  SumDOutMin=[]  SumDOutMax=[]  DifferentiatorOutMin=[]  DifferentiatorOutMax=[]  FilterDiffOutCoefMin=[]  FilterDiffOutCoefMax=[]  ReciprocalOutMin=[]  ReciprocalOutMax=[]  SumDenOutMin=[]  SumDenOutMax=[]  SumNumOutMin=[]  SumNumOutMax=[]  DivideOutMin=[]  DivideOutMax=[]  UdiffTsProdOutMin=[]  UdiffTsProdOutMax=[]  NTsProdOutMin=[]  NTsProdOutMax=[]  UintegralTsProdOutMin=[]  UintegralTsProdOutMax=[]  UngainTsProdOutMin=[]  UngainTsProdOutMax=[]  ClampingZeroOutDataTypeStr=Inherit: Inherit via back propagation  ClampingZeroOutMin=[]  ClampingZeroOutMax=[]  FilterDenConstantOutDataTypeStr=Inherit: Inherit via back propagation  FilterDenConstantOutMin=[]  FilterDenConstantOutMax=[]  PCopyOutDataTypeStr=Inherit: Inherit via back propagation  PCopyOutMin=[]  PCopyOutMax=[]  NCopyOutDataTypeStr=Inherit: Inherit via back propagation  NCopyOutMin=[]  NCopyOutMax=[]  IntegratorContinuousStateAttributes=''  IntegratorStateMustResolveToSignalObject=off  IntegratorRTWStateStorageClass=Auto  FilterContinuousStateAttributes=''  FilterStateMustResolveToSignalObject=off  FilterRTWStateStorageClass=Auto  ParallelPVariant=InternalParameters  IdealPVariant=Disabled  IVariant=InternalParameters  DVariant=InternalParameters  IntegratorVariant=Continuous  SatVariant=Disabled  AWVariant=Passthrough  PCopyVariant=Disabled  TRVariant=Disabled  FdbkBlocksVariant=Forward  IdealPFdbkVariant=Disabled  SatFdbkVariant=Disabled  DerivativeFilterVariant=ContFilter  NVariant=InternalParameters  NCopyVariant=Disabled  FilterICVariant=InternalICsFilter  IntegratorICVariant=InternalICs  ExternalResetVariant=Disabled  TRSumVariant=Passthrough  SumFdbkVariant=Disabled  SumVariant=Sum_PID  TsampFilterVariant=InternalTs  TsampNgainVariant=Passthrough  TsampIntegralVariant=Disabled_SignalSpec  ExternalSaturationOutDataTypeStr=Inherit: Same as second input  DerivativeSourceVariant=ErrorSignal
  Reshape : Reshape
  Signal Copy : SignalConversion  OverrideOpt=off
  Sum : Sum  Inputs=|+-
  Sum1 : Sum  Inputs=|-+
  AccelAndOmegadot_Reaug : Outport
  log : Outport  Port=2
  wires:
  Matrix Concatenate/1 -> Reshape/1
  Sys_input/1 -> Bus Selector1/1, Bus Selector3/1
  Bus Creator/1 -> log/1
  PID Controller/1 -> Matrix Concatenate/1  "Accel"
  Reshape/1 -> AccelAndOmegadot_Reaug/1
  Bus Selector4/1 -> Matrix Multiply/1  "<DCM_NED2Body>"
  Bus Selector3/1 -> Matrix Multiply/2  "<ned_vel_mps>"
  DCMs/1 -> Bus Selector4/1
  Matrix Multiply/1 -> Sum/2, Bus Creator/3  "uvw_mps"
  Bus Selector1/1 -> Signal Copy/1  "<gyro_radps>"
  uvw_cmds_mps/1 -> Cast To Single/1
  body_rot_rate_cmds_rps/1 -> Cast To Single1/1
  Cast To Single/1 -> [uvw_cmds_mps], Sum/1  "uvw_cmds_mps"
  Cast To Single1/1 -> [body_rot_rate_cmds_rps], Sum1/2  "body_rot_rate_cmds_rps"
  Signal Copy/1 -> Bus Creator/5, Sum1/1  "body_rot_rate_rps"
  Sum/1 -> Bus Creator/2, Cast To Double/1  "uvw_err_mps"
  Sum1/1 -> Bus Creator/6, Cast To Double1/1  "body_rot_rate_err_rps"
  PID Controller1/1 -> Matrix Concatenate/2  "Omegadot"
  Cast To Double/1 -> PID Controller/1
  Cast To Double1/1 -> PID Controller1/1
  [uvw_cmds_mps] -> Bus Creator/1
  [body_rot_rate_cmds_rps] -> Bus Creator/4

== system seldom/cmd to raw pwm ==
  ramp_completed : Inport
  pwm_cmd : Inport  Port=2
  Constant : Constant  Value=zeros(1,Aircraft.Motor.nMotor)  OutDataTypeStr=single
  Data Type Conversion : DataTypeConversion  OutDataTypeStr=int16  SaturateOnIntegerOverflow=off  RndMeth=Floor
  NOT : Logic  Operator=NOT  IconShape=distinctive  AllPortsSameDT=off  OutDataTypeStr=boolean
  Switch : Switch  Criteria=u2 > Threshold  SaturateOnIntegerOverflow=off  InputSameDT=off
  motor_PWM_denormalize : Subsystem
  motor_PWM_denormalize1 : Subsystem
  PwmCmd : Outport
  wires:
  Switch/1 -> Data Type Conversion/1
  motor_PWM_denormalize/1(raw_output) -> Switch/1
  pwm_cmd/1 -> motor_PWM_denormalize/1(normalized_input)
  Constant/1 -> motor_PWM_denormalize1/1(normalized_input)
  Data Type Conversion/1 -> PwmCmd/1  "cnt"
  ramp_completed/1 -> NOT/1
  NOT/1 -> Switch/2
  motor_PWM_denormalize1/1(raw_output) -> Switch/3

== system seldom/emergency_stop_system ==
  input_signal : Inport
  emmergency_stop_signal : Inport  Port=2
  Constant : Constant  Value=zeros(1,Aircraft.Motor.nMotor)  VectorParams1D=off  OutDataTypeStr=single
  emergency_switch : Switch  Criteria=u2 > Threshold  Threshold=0.5  SaturateOnIntegerOverflow=off  InputSameDT=off
  pwm_cmd : Outport
  wires:
  emergency_switch/1 -> pwm_cmd/1
  emmergency_stop_signal/1 -> emergency_switch/2
  Constant/1 -> emergency_switch/1
  input_signal/1 -> emergency_switch/3

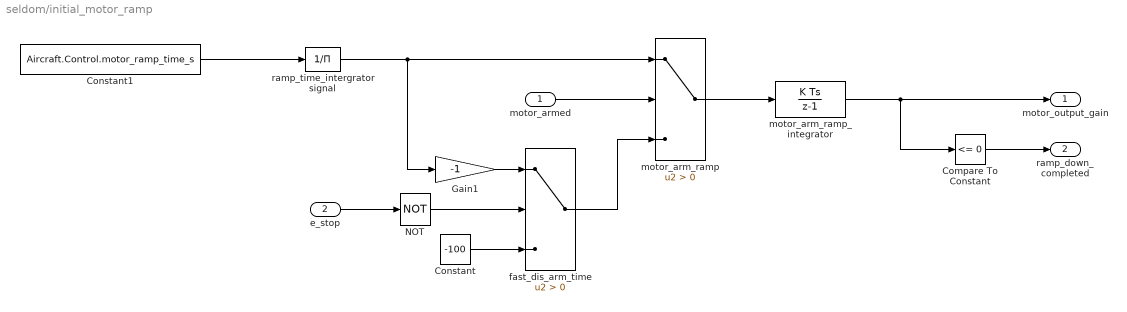
== system seldom/initial_motor_ramp ==
  motor_armed : Inport
  e_stop : Inport  Port=2
  Compare To Constant : simulink/Logic and Bit Operations/Compare To Constant  relop=<=  const=0  OutDataTypeStr=boolean
  Constant : Constant  Value=-100  OutDataTypeStr=single
  Constant1 : Constant  Value=Aircraft.Control.motor_ramp_time_s  OutDataTypeStr=single
  Gain1 : Gain  Gain=-1
  NOT : Logic  Operator=NOT  IconShape=distinctive  AllPortsSameDT=off  OutDataTypeStr=boolean
  fast_dis_arm_time : Switch  Criteria=u2 > Threshold  SaturateOnIntegerOverflow=off  InputSameDT=off
  motor_arm_ramp : Switch  Criteria=u2 > Threshold  SaturateOnIntegerOverflow=off  InputSameDT=off
  motor_arm_ramp_integrator : DiscreteIntegrator  SampleTime=framePeriod_s  LimitOutput=on  UpperSaturationLimit=1  LowerSaturationLimit=0  ICPrevOutput=DiscIntNeverNeededParam  ICPrevScaledInput=DiscIntNeverNeededParam
  ramp_time_intergrator signal : Product  Inputs=/
  motor_output_gain : Outport
  ramp_down_completed : Outport  Port=2
  wires:
  Constant1/1 -> ramp_time_intergrator signal/1
  motor_arm_ramp/1 -> motor_arm_ramp_integrator/1
  ramp_time_intergrator signal/1 -> Gain1/1, motor_arm_ramp/1
  motor_arm_ramp_integrator/1 -> motor_output_gain/1, Compare To Constant/1
  motor_armed/1 -> motor_arm_ramp/2
  e_stop/1 -> NOT/1
  NOT/1 -> fast_dis_arm_time/2
  fast_dis_arm_time/1 -> motor_arm_ramp/3
  Gain1/1 -> fast_dis_arm_time/1
  Constant/1 -> fast_dis_arm_time/3
  Compare To Constant/1 -> ramp_down_completed/1

== system seldom/CmdSelection/e_stop_norm ==
  raw_sbus_in : Inport
  Constant : Constant  Value=172  OutDataTypeStr=single
  Constant1 : Constant  Value=-1  OutDataTypeStr=single
  Constant2 : Constant  OutDataTypeStr=single
  Constant3 : Constant  Value=1811  OutDataTypeStr=single
  remap : MATLAB Function  TreatAsAtomicUnit=on
  normalized_out : Outport
  wires:
  Constant2/1 -> remap/5(out_max)
  Constant1/1 -> remap/4(out_min)
  Constant3/1 -> remap/3(in_max)
  Constant/1 -> remap/2(in_min)
  remap/1(norm_out) -> normalized_out/1
  raw_sbus_in/1 -> remap/1(raw_in)

== system seldom/CmdSelection/mode_norm ==
  raw_sbus_in : Inport
  Constant : Constant  Value=172  OutDataTypeStr=single
  Constant1 : Constant  Value=0  OutDataTypeStr=single
  Constant2 : Constant  Value=2  OutDataTypeStr=single
  Constant3 : Constant  Value=1811  OutDataTypeStr=single
  remap : MATLAB Function  TreatAsAtomicUnit=on
  normalized_out : Outport
  wires:
  raw_sbus_in/1 -> remap/1(raw_in)
  remap/1(norm_out) -> normalized_out/1
  Constant/1 -> remap/2(in_min)
  Constant3/1 -> remap/3(in_max)
  Constant1/1 -> remap/4(out_min)
  Constant2/1 -> remap/5(out_max)

== system seldom/CmdSelection/pitch_norm_deadband ==
  raw_sbus_in : Inport
  deadband : Inport  Port=2
  Constant : Constant  Value=172  OutDataTypeStr=single
  Constant1 : Constant  Value=-1  OutDataTypeStr=single
  Constant2 : Constant  OutDataTypeStr=single
  Constant3 : Constant  Value=1811  OutDataTypeStr=single
  remap_with_deadband : MATLAB Function  TreatAsAtomicUnit=on
  normalized_out : Outport
  wires:
  raw_sbus_in/1 -> remap_with_deadband/1(raw_in)
  remap_with_deadband/1(norm_out) -> normalized_out/1
  Constant/1 -> remap_with_deadband/2(in_min)
  Constant3/1 -> remap_with_deadband/3(in_max)
  Constant1/1 -> remap_with_deadband/4(out_min)
  Constant2/1 -> remap_with_deadband/5(out_max)
  deadband/1 -> remap_with_deadband/6(deadband)

== system seldom/CmdSelection/roll_norm_deadband ==
  raw_sbus_in : Inport
  deadband : Inport  Port=2
  Constant : Constant  Value=172  OutDataTypeStr=single
  Constant1 : Constant  Value=-1  OutDataTypeStr=single
  Constant2 : Constant  OutDataTypeStr=single
  Constant3 : Constant  Value=1811  OutDataTypeStr=single
  remap_with_deadband : MATLAB Function  TreatAsAtomicUnit=on
  normalized_out : Outport
  wires:
  raw_sbus_in/1 -> remap_with_deadband/1(raw_in)
  remap_with_deadband/1(norm_out) -> normalized_out/1
  Constant/1 -> remap_with_deadband/2(in_min)
  Constant3/1 -> remap_with_deadband/3(in_max)
  Constant1/1 -> remap_with_deadband/4(out_min)
  Constant2/1 -> remap_with_deadband/5(out_max)
  deadband/1 -> remap_with_deadband/6(deadband)

== system seldom/CmdSelection/vel_E_cmd_fps_norm_deadband ==
  raw_sbus_in : Inport
  deadband : Inport  Port=2
  Constant : Constant  Value=172  OutDataTypeStr=single
  Constant1 : Constant  Value=-1  OutDataTypeStr=single
  Constant2 : Constant  OutDataTypeStr=single
  Constant3 : Constant  Value=1811  OutDataTypeStr=single
  remap_with_deadband : MATLAB Function  TreatAsAtomicUnit=on
  normalized_out : Outport
  wires:
  deadband/1 -> remap_with_deadband/6(deadband)
  Constant2/1 -> remap_with_deadband/5(out_max)
  Constant1/1 -> remap_with_deadband/4(out_min)
  Constant3/1 -> remap_with_deadband/3(in_max)
  Constant/1 -> remap_with_deadband/2(in_min)
  remap_with_deadband/1(norm_out) -> normalized_out/1
  raw_sbus_in/1 -> remap_with_deadband/1(raw_in)

== system seldom/CmdSelection/vel_N_cmd_fps_norm_deadband ==
  raw_sbus_in : Inport
  deadband : Inport  Port=2
  Constant : Constant  Value=172  OutDataTypeStr=single
  Constant1 : Constant  Value=-1  OutDataTypeStr=single
  Constant2 : Constant  OutDataTypeStr=single
  Constant3 : Constant  Value=1811  OutDataTypeStr=single
  remap_with_deadband : MATLAB Function  TreatAsAtomicUnit=on
  normalized_out : Outport
  wires:
  raw_sbus_in/1 -> remap_with_deadband/1(raw_in)
  remap_with_deadband/1(norm_out) -> normalized_out/1
  Constant/1 -> remap_with_deadband/2(in_min)
  Constant3/1 -> remap_with_deadband/3(in_max)
  Constant1/1 -> remap_with_deadband/4(out_min)
  Constant2/1 -> remap_with_deadband/5(out_max)
  deadband/1 -> remap_with_deadband/6(deadband)

== system seldom/CmdSelection/vel_U_cmd_fps_norm_deadband ==
  raw_sbus_in : Inport
  deadband : Inport  Port=2
  Constant : Constant  Value=172  OutDataTypeStr=single
  Constant1 : Constant  Value=-1  OutDataTypeStr=single
  Constant2 : Constant  OutDataTypeStr=single
  Constant3 : Constant  Value=1811  OutDataTypeStr=single
  remap_with_deadband : MATLAB Function  TreatAsAtomicUnit=on
  normalized_out : Outport
  wires:
  deadband/1 -> remap_with_deadband/6(deadband)
  Constant2/1 -> remap_with_deadband/5(out_max)
  Constant1/1 -> remap_with_deadband/4(out_min)
  Constant3/1 -> remap_with_deadband/3(in_max)
  Constant/1 -> remap_with_deadband/2(in_min)
  remap_with_deadband/1(norm_out) -> normalized_out/1
  raw_sbus_in/1 -> remap_with_deadband/1(raw_in)

== system seldom/CmdSelection/yaw_norm_deadband ==
  raw_sbus_in : Inport
  deadband : Inport  Port=2
  Constant : Constant  Value=172  OutDataTypeStr=single
  Constant1 : Constant  Value=-1  OutDataTypeStr=single
  Constant2 : Constant  OutDataTypeStr=single
  Constant3 : Constant  Value=1811  OutDataTypeStr=single
  remap_with_deadband : MATLAB Function  TreatAsAtomicUnit=on
  normalized_out : Outport
  wires:
  raw_sbus_in/1 -> remap_with_deadband/1(raw_in)
  remap_with_deadband/1(norm_out) -> normalized_out/1
  Constant/1 -> remap_with_deadband/2(in_min)
  Constant3/1 -> remap_with_deadband/3(in_max)
  Constant1/1 -> remap_with_deadband/4(out_min)
  Constant2/1 -> remap_with_deadband/5(out_max)
  deadband/1 -> remap_with_deadband/6(deadband)

== system seldom/Deaug/AeroDeaug ==
  note: Deaugmentation for deceleration due to drag and rotational deceleration due to dynamic derivatives.
      |
      | For the moments, should just be able to dimensionalize Cl_p, Cm_q, and Cn_r then multiply by p, q, and r respectively to get the moments applied. Finally divide by Ixx, Iyy, Izz respectively to get angular accelerations that we need to deaugment.
      |
      | Similarly for the forces, should be able to dimensionalize CD to get the force applied. Next divide by mass to get acceleration this will cause. Finally, based on velocity vector orientation in the body frame, distribute this to udot, vdot, and wdot to get accelerations that we need to deaugment.
  omega : Inport
  uvw : Inport  Port=2
  Mux1 : Mux  Inputs=6
  Terminator : Terminator
  Terminator1 : Terminator
  AeroDeaug : Outport
  wires:
  omega/1 -> Terminator/1
  Mux1/1 -> AeroDeaug/1  "AeroDeaug"
  uvw/1 -> Terminator1/1
  ? -> Mux1/1  "udot"
  ? -> Mux1/2  "vdot"
  ? -> Mux1/3  "wdot"
  ? -> Mux1/4  "pdot"
  ? -> Mux1/5  "qdot"
  ? -> Mux1/6  "rdot"

== system seldom/Deaug/GravityVectorCompensation ==
  note: No angular acceleration (omegadot) from gravity since it acts at the CG.
  DCM_LocalNav2Body : Inport
  LLA : Inport  Port=2
  Constant1 : Constant  Value=0
  Demux : Demux  Outputs=3
  Matrix Multiply : Product  Multiplication=Matrix(*)
  Mux1 : Mux  Inputs=6
  "WGS84 Gravity Model  " : GravityWGS84
  AccelAndOmegadot_grav_body : Outport
  wires:
  DCM_LocalNav2Body/1 -> Matrix Multiply/1
  Matrix Multiply/1 -> Demux/1  "accel_grav_body"
  LLA/1 -> "WGS84 Gravity Model  "/1
  "WGS84 Gravity Model  "/1 -> Matrix Multiply/2  "gravity_NED"
  Mux1/1 -> AccelAndOmegadot_grav_body/1
  Demux/1 -> Mux1/1
  Demux/2 -> Mux1/2
  Demux/3 -> Mux1/3
  Constant1/1 -> Mux1/5, Mux1/6, Mux1/4

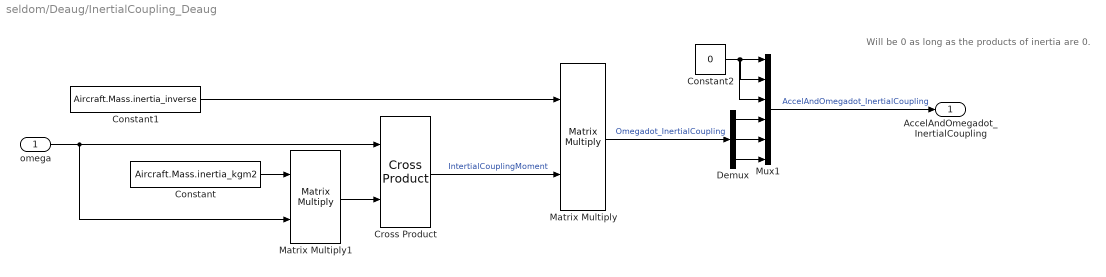
== system seldom/Deaug/InertialCoupling_Deaug ==
  note: Will be 0 as long as the products of inertia are 0.
  omega : Inport
  Constant : Constant  Value=Aircraft.Mass.inertia_kgm2
  Constant1 : Constant  Value=Aircraft.Mass.inertia_inverse
  Constant2 : Constant  Value=0
  Cross Product : matrix_library/Cross Product
  Demux : Demux  Outputs=3
  Matrix Multiply : Product  Multiplication=Matrix(*)
  Matrix Multiply1 : Product  Multiplication=Matrix(*)
  Mux1 : Mux  Inputs=6
  AccelAndOmegadot_InertialCoupling : Outport
  wires:
  Mux1/1 -> AccelAndOmegadot_InertialCoupling/1  "AccelAndOmegadot_InertialCoupling"
  Constant1/1 -> Matrix Multiply/1
  omega/1 -> Matrix Multiply1/2, Cross Product/1
  Cross Product/1 -> Matrix Multiply/2  "IntertialCouplingMoment"
  Constant/1 -> Matrix Multiply1/1
  Matrix Multiply1/1 -> Cross Product/2
  Demux/1 -> Mux1/4
  Demux/2 -> Mux1/5
  Demux/3 -> Mux1/6
  Constant2/1 -> Mux1/3, Mux1/2, Mux1/1
  Matrix Multiply/1 -> Demux/1  "Omegadot_InertialCoupling"

== system seldom/EmergencyStopping/Subsystem ==
  <e_stop> : Inport
  Abs1 : Abs  SaturateOnIntegerOverflow=off
  Compare To Constant : simulink/Logic and Bit Operations/Compare To Constant  relop=>=  const=0.98  OutDataTypeStr=boolean
  e_stop counter : Subsystem
  e_stop_filtered : Outport
  wires:
  Compare To Constant/1 -> e_stop counter/Enable
  Abs1/1 -> Compare To Constant/1
  <e_stop>/1 -> e_stop counter/1(motor_e_stop_raw), Abs1/1
  e_stop counter/1(e_stop_filtered) -> e_stop_filtered/1

== system seldom/EmergencyStopping/Subsystem1 ==
  <inceptor_health> : Inport
  Add : Sum
  Cast To Single : DataTypeConversion  OutDataTypeStr=single  SaturateOnIntegerOverflow=off  RndMeth=Floor
  Constant : Constant  Value=-0.5
  Gain : Gain  Gain=2
  Subsystem : Subsystem
  inceptor_health_filtered : Outport
  wires:
  Subsystem/1(incept_health_filter) -> inceptor_health_filtered/1
  <inceptor_health>/1 -> Cast To Single/1
  Cast To Single/1 -> Add/1
  Constant/1 -> Add/2
  Gain/1 -> Subsystem/1(<incept_health_raw>)
  Add/1 -> Gain/1

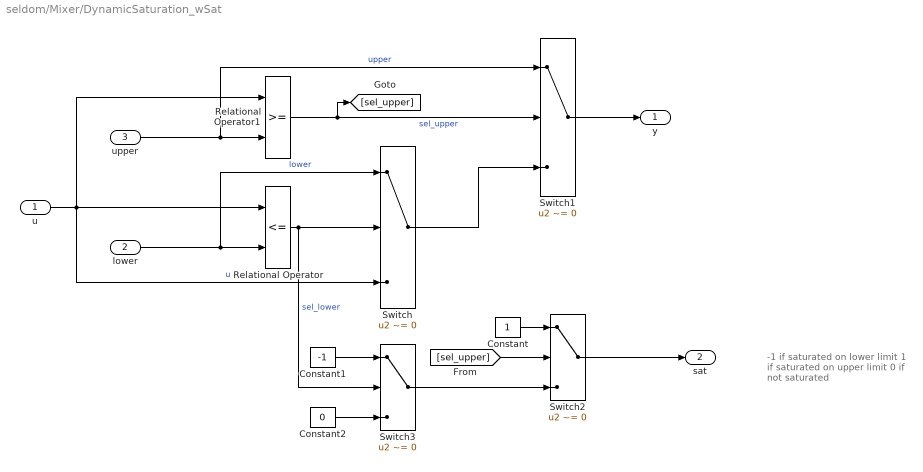
== system seldom/Mixer/DynamicSaturation_wSat ==
  note: -1 if saturated on lower limit
      | 1 if saturated on upper limit
      | 0 if not saturated
  u : Inport
  lower : Inport  Port=2
  upper : Inport  Port=3
  Constant : Constant
  Constant1 : Constant  Value=-1
  Constant2 : Constant  Value=0
  Relational Operator : RelationalOperator  Operator=<=  OutDataTypeStr=boolean  RndMeth=Simplest  InputSameDT=off
  Relational Operator1 : RelationalOperator  OutDataTypeStr=boolean  RndMeth=Simplest  InputSameDT=off
  Switch{,1..3} (4 alike) : Switch  Criteria=u2 ~= 0  SaturateOnIntegerOverflow=off  InputSameDT=off
  y : Outport
  sat : Outport  Port=2
  wires:
  Relational Operator/1 -> Switch3/2, Switch/2  "sel_lower"
  lower/1 -> Switch/1, Relational Operator/2  "lower"
  u/1 -> Relational Operator1/1, Switch/3, Relational Operator/1  "u"
  Relational Operator1/1 -> [sel_upper], Switch1/2  "sel_upper"
  upper/1 -> Switch1/1, Relational Operator1/2  "upper"
  Switch/1 -> Switch1/3
  Switch1/1 -> y/1
  Switch2/1 -> sat/1
  Switch3/1 -> Switch2/3
  Constant/1 -> Switch2/1
  Constant1/1 -> Switch3/1
  Constant2/1 -> Switch3/3
  [sel_upper] -> Switch2/2

== system seldom/Mixer/LogicalLatchNonResettable ==
  u : Inport
  Logical Operator : Logic  Operator=OR  AllPortsSameDT=off  OutDataTypeStr=boolean
  Memory : Memory  InitialCondition=false  InheritSampleTime=on
  y : Outport
  wires:
  u/1 -> Logical Operator/1
  Memory/1 -> Logical Operator/2
  Logical Operator/1 -> Memory/1, y/1

== system seldom/cmd to raw pwm/motor_PWM_denormalize ==
  normalized_input : Inport
  Constant : Constant  Value=Aircraft.PWM.norm_min  OutDataTypeStr=single
  Constant1 : Constant  Value=Aircraft.PWM.min  OutDataTypeStr=single
  Constant2 : Constant  Value=Aircraft.PWM.max  OutDataTypeStr=single
  Constant3 : Constant  Value=Aircraft.PWM.norm_max  OutDataTypeStr=single
  remap : MATLAB Function  TreatAsAtomicUnit=on
  raw_output : Outport
  wires:
  Constant2/1 -> remap/5(out_max)
  Constant1/1 -> remap/4(out_min)
  Constant3/1 -> remap/3(in_max)
  Constant/1 -> remap/2(in_min)
  remap/1(raw_out) -> raw_output/1
  normalized_input/1 -> remap/1(norm_in)

== system seldom/cmd to raw pwm/motor_PWM_denormalize1 ==
  normalized_input : Inport
  Constant : Constant  Value=Aircraft.PWM.norm_min  OutDataTypeStr=single
  Constant1 : Constant  Value=Aircraft.PWM.min  OutDataTypeStr=single
  Constant2 : Constant  Value=Aircraft.PWM.max  OutDataTypeStr=single
  Constant3 : Constant  Value=Aircraft.PWM.norm_max  OutDataTypeStr=single
  remap : MATLAB Function  TreatAsAtomicUnit=on
  raw_output : Outport
  wires:
  normalized_input/1 -> remap/1(norm_in)
  remap/1(raw_out) -> raw_output/1
  Constant/1 -> remap/2(in_min)
  Constant3/1 -> remap/3(in_max)
  Constant1/1 -> remap/4(out_min)
  Constant2/1 -> remap/5(out_max)
